simulink model "hydroplane"  (R2020b)
settings: Solver=VariableStepAuto  StartTime=0.0  StopTime=10.0  RelTol=1e-3
model workspace (MAT data in the model file):
  F = 1
settings Model: Creator=divyaprakash  LastModifiedBy=divyaprakash

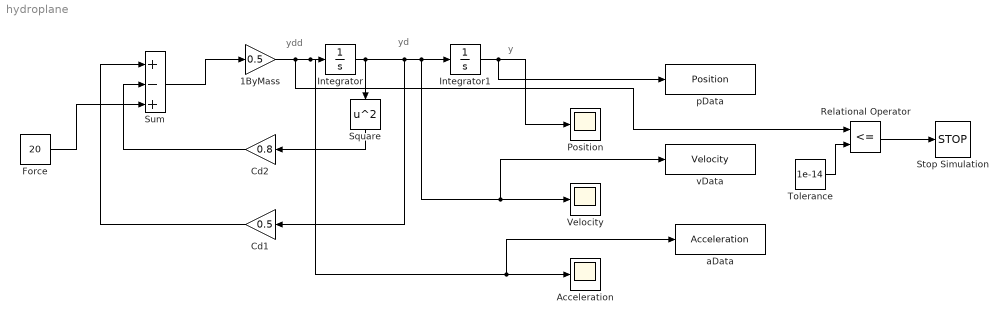
== system hydroplane ==
  note: y
  note: yd
  note: ydd
  1ByMass : Gain  Gain=0.5
  Acceleration : Scope
  Cd1 : Gain  Gain=0.5
  Cd2 : Gain  Gain=0.8
  Force : Constant  Value=20
  Integrator : Integrator
  Integrator1 : Integrator
  Position : Scope
  Relational Operator : RelationalOperator  Operator=<=  OutDataTypeStr=boolean  RndMeth=Simplest
  Square : Math  Operator=square  SaturateOnIntegerOverflow=on
  Stop Simulation : Stop
  Sum : Sum  Inputs=|+-+
  Tolerance : Constant  Value=1e-14
  Velocity : Scope
  aData : ToWorkspace  VariableName=Acceleration  SaveFormat=Timeseries  SampleTime=-1
  pData : ToWorkspace  VariableName=Position  SaveFormat=Timeseries  SampleTime=-1
  vData : ToWorkspace  VariableName=Velocity  SaveFormat=Timeseries  SampleTime=-1
  wires:
  Integrator/1 -> Cd1/1, vData/1, Velocity/1, Integrator1/1, Square/1
  Integrator1/1 -> pData/1, Position/1
  1ByMass/1 -> Relational Operator/1, aData/1, Acceleration/1, Integrator/1
  Sum/1 -> 1ByMass/1
  Cd2/1 -> Sum/2
  Cd1/1 -> Sum/1
  Force/1 -> Sum/3
  Square/1 -> Cd2/1
  Tolerance/1 -> Relational Operator/2
  Relational Operator/1 -> Stop Simulation/1
